simulink model "ReactionWheelControl"  (R2024a)
settings: Solver=VariableStepAuto  StartTime=0.0  StopTime=10.0  RelTol=1e-3
values from neighbouring files (symbols this model uses):
  I = diag([m*(y^2+z^2);            m*(x^2+z^2);            m*(x^2+y^2)])    [aero421_finalProject.m]    (also in aero421_finalProject_D.m)
settings Model: Creator=joels  LastModifiedBy=joels

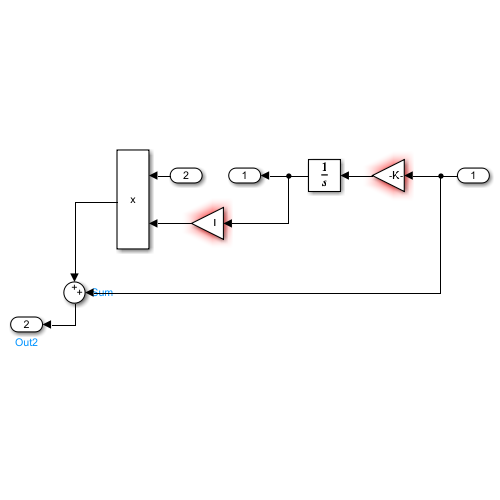
[thumbnail: Simulink's stored preview of the top-level diagram]
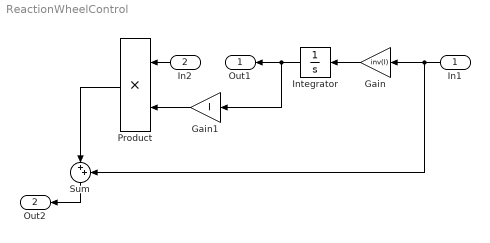
== system ReactionWheelControl ==
  In1 : Inport
  In2 : Inport  Port=2
  Gain : Gain  Gain=inv(I)
  Gain1 : Gain  Gain=I
  Integrator : Integrator
  Product : Product
  Sum : Sum  Inputs=|++
  Out1 : Outport
  Out2 : Outport  Port=2
  wires:
  In1/1 -> Sum/2, Gain/1
  Gain/1 -> Integrator/1
  Integrator/1 -> Gain1/1, Out1/1
  Gain1/1 -> Product/2
  In2/1 -> Product/1
  Product/1 -> Sum/1
  Sum/1 -> Out2/1
